simulink model "communicationCPU2_controller1"  (R2020a)
settings: Solver=FixedStepAuto  StartTime=0.0  StopTime=Inf  RelTol=1e-3  EnableMultiTasking=on
InitFcn:
  | Send_PSO_sample_time = 0.1;
undefined symbols (not defined in the file): C28x, CPU1, CPU2
libraries: c280xlib x10, c2837xDlib x3
settings Model: SimulationMode=external  ExtModeTrigDuration=8  Creator=Jason  LastModifiedBy=Jason
settings SolverCC: AutoInsertRateTranBlk=on
settings OptimizationCC: DefaultUnderspecifiedDataType=single  EnhancedBackFolding=on  PassReuseOutputArgsAs=Individual arguments  MaxStackSize=1024  OptimizeBlockOrder=speed  DifferentSizesBufferReuse=on  OptimizationCustomize=off  DenormalBehavior=FlushToZero  EfficientTunableParamExpr=on
settings DebuggingCC: ParameterTunabilityLossMsg=error
settings HardwareCC: ProdBitPerChar=16  ProdBitPerInt=16  ProdBitPerPointer=32  ProdBitPerSizeT=32  ProdBitPerPtrDiffT=32  ProdLargestAtomicInteger=Integer  ProdLargestAtomicFloat=None  ProdWordSize=16  ProdLongLongMode=on  ProdHWDeviceType=Texas Instruments->C2000
settings RTWCC: SystemTargetFile=ert.tlc  HardwareBoard=TI Delfino F28379D LaunchPad  TLCOptions=-aInlineSetEventsForThisBaseRateFcn=TLC_FALSE -aSuppressMultiTaskScheduler=TLC_FALSE -aRateBasedStepFcn=1  TemplateMakefile=ert_default_tmf  Toolchain=Texas Instruments Code Composer Studio (C2000)
settings CodeAppCC: ForceParamTrailComments=on  IgnoreCustomStorageClasses=off  OperatorAnnotations=on  SimulinkDataObjDesc=on  SFDataObjDesc=on  InsertBlockDesc=on
settings ERTTargetCC: TargetLangStandard=C99 (ISO)  CodeReplacementLibrary=TI C28x  SupportVariableSizeSignals=on  ExtModeStaticAllocSize=10000

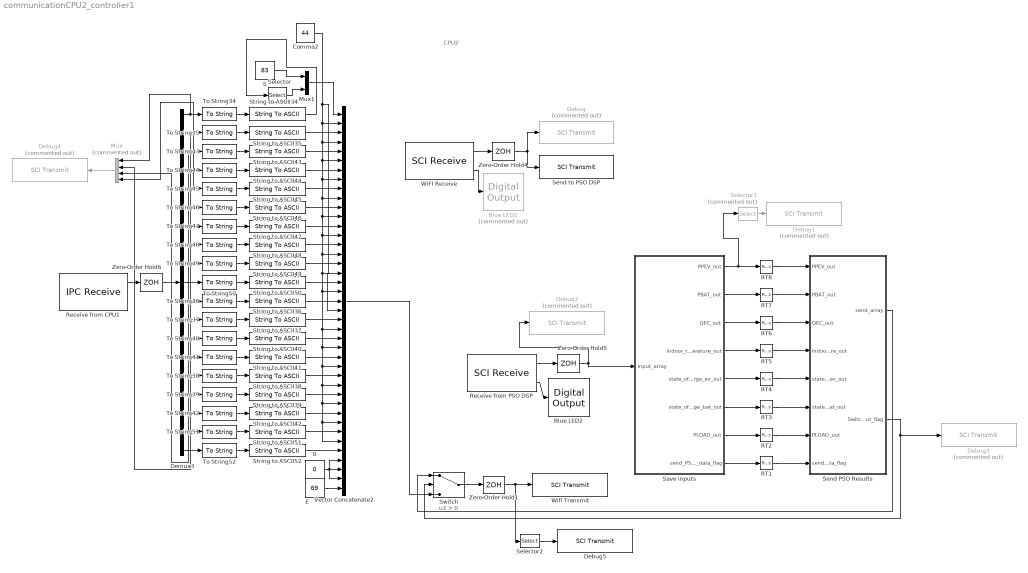
== system communicationCPU2_controller1 ==
  note: CPU2
  0 : Constant  Value=0  OutDataTypeStr=uint8  SampleTime=-1
  Blue LED1 : c2837xDlib/Digital Output  Commented=on  GPIO_Number=GPIO24~GPIO31  GPIO_Bit0=off  GPIO_BIT0_Toggle=off  GPIO_Bit1=off  GPIO_BIT1_Toggle=off  GPIO_Bit2=off  GPIO_BIT2_Toggle=off  GPIO_Bit3=off  GPIO_BIT3_Toggle=off  GPIO_Bit4=off  GPIO_BIT4_Toggle=off  GPIO_Bit5=off  GPIO_BIT5_Toggle=off  GPIO_Bit6=off  GPIO_BIT6_Toggle=off  GPIO_Bit7=on  GPIO_BIT7_Toggle=off
      settings: SourceProductBaseCode=TIC2000
  Blue LED2 : c2837xDlib/Digital Output  GPIO_Number=GPIO24~GPIO31  GPIO_Bit0=off  GPIO_BIT0_Toggle=off  GPIO_Bit1=off  GPIO_BIT1_Toggle=off  GPIO_Bit2=off  GPIO_BIT2_Toggle=off  GPIO_Bit3=off  GPIO_BIT3_Toggle=off  GPIO_Bit4=off  GPIO_BIT4_Toggle=off  GPIO_Bit5=off  GPIO_BIT5_Toggle=off  GPIO_Bit6=off  GPIO_BIT6_Toggle=off  GPIO_Bit7=on  GPIO_BIT7_Toggle=off
      settings: SourceProductBaseCode=TIC2000
  Comma2 : Constant  Value=44  OutDataTypeStr=uint8  SampleTime=-1
  Debug{,1..4} (5 alike) : c280xlib/SCI Transmit  Commented=on  sciModule=A  dataHead=''  dataTail=''  postInterrupt=off  numFifo=1
  Debug5 : c280xlib/SCI Transmit  sciModule=A  dataHead=''  dataTail=''  postInterrupt=off  numFifo=1
  Demux3 : Demux  Outputs=19
  E : Constant  Value=69  OutDataTypeStr=uint8  SampleTime=-1
  Mux : Mux  Commented=on
  Mux1 : Mux  Inputs=2
  RT{1..8} (8 alike) : RateTransition  OutPortSampleTime=Send_PSO_sample_time
  Receive from CPU1 : c2837xDlib/IPC Receive  blkParamProc=F2837x  SelectSource=C28x (CPU1/CPU2)  SelectChannel=0  DataType=single  DataLength=19  EnableBlocking=off  SampleTime=0.5
      settings: SourceProductBaseCode=TIC2000
  Receive from PSO DSP : c280xlib/SCI Receive  sciModule=B  dataHead=''  dataTail=''  dataType=uint8  dataDim=10  initValue=66  errOption=Output the last received value  errValue=0  sampleTime=0.005  outputStatus=on  postInterrupt=off  numFifo=1
      settings: SourceProductBaseCode=TIC2000
  S : Constant  Value=83  OutDataTypeStr=uint8  SampleTime=-1
  Save inputs : MATLAB Function  TreatAsAtomicUnit=on
  Selector : Selector  InputPortWidth=12  IndexOptions=Index vector (dialog)  Indices=[2:12]  OutputSizes=1
  Selector1 : Selector  Commented=on  InputPortWidth=500  IndexOptions=Index vector (dialog)  Indices=[481:500]  OutputSizes=1
  Selector2 : Selector  InputPortWidth=250  IndexOptions=Index vector (dialog)  Indices=[1:11]  OutputSizes=1
  Send PSO Results : MATLAB Function  TreatAsAtomicUnit=on
  Send to PSO DSP : c280xlib/SCI Transmit  sciModule=B  dataHead=''  dataTail=''  postInterrupt=off  numFifo=1
  String to ASCII{34..52} (19 alike) : StringToASCII  OutputVectorSize=12
  Switch : Switch  Criteria=u2 > Threshold
  To String{34..52} (19 alike) : ToString
  Vector Concatenate2 : Concatenate  NumInputs=41
  WiFI Receive : c280xlib/SCI Receive  sciModule=C  dataHead=''  dataTail=''  dataType=uint8  dataDim=11  initValue=50  errOption=Output the last received value  errValue=0  sampleTime=0.005  outputStatus=on  postInterrupt=off  numFifo=1
      settings: SourceProductBaseCode=TIC2000
  Wifi Transmit : c280xlib/SCI Transmit  sciModule=C  dataHead=''  dataTail=''  postInterrupt=off  numFifo=1
  Zero-Order Hold1 : ZeroOrderHold  SampleTime=0.4
  Zero-Order Hold4 : ZeroOrderHold  SampleTime=0.1
  Zero-Order Hold5 : ZeroOrderHold  SampleTime=0.05
  Zero-Order Hold6 : ZeroOrderHold  SampleTime=0.1
  wires:
  Demux3/2 -> Mux/2, To String35/1
  String to ASCII48/1 -> Vector Concatenate2/15
  To String39/1 -> String to ASCII39/1
  To String38/1 -> String to ASCII38/1
  String to ASCII39/1 -> Vector Concatenate2/31
  Demux3/17 -> To String42/1
  Demux3/16 -> To String39/1
  To String42/1 -> String to ASCII42/1
  Demux3/10 -> To String50/1
  Demux3/12 -> To String37/1
  Demux3/15 -> To String38/1
  String to ASCII35/1 -> Vector Concatenate2/3
  String to ASCII38/1 -> Vector Concatenate2/29
  String to ASCII42/1 -> Vector Concatenate2/33
  Demux3/14 -> To String41/1
  String to ASCII50/1 -> Vector Concatenate2/19
  String to ASCII44/1 -> Vector Concatenate2/7
  String to ASCII49/1 -> Vector Concatenate2/17
  String to ASCII40/1 -> Vector Concatenate2/25
  To String37/1 -> String to ASCII37/1
  To String36/1 -> String to ASCII36/1
  To String50/1 -> String to ASCII50/1
  String to ASCII46/1 -> Vector Concatenate2/11
  Demux3/8 -> To String48/1
  Demux3/7 -> To String47/1
  Demux3/6 -> To String46/1
  To String35/1 -> String to ASCII35/1
  To String47/1 -> String to ASCII47/1
  To String48/1 -> String to ASCII48/1
  String to ASCII36/1 -> Vector Concatenate2/21
  Demux3/5 -> Mux/4, To String45/1
  To String41/1 -> String to ASCII41/1
  Comma2/1 -> Vector Concatenate2/14, Vector Concatenate2/34, Vector Concatenate2/36, Vector Concatenate2/32, Vector Concatenate2/30, Vector Concatenate2/28, Vector Concatenate2/26, Vector Concatenate2/24, Vector Concatenate2/22, Vector Concatenate2/20, Vector Concatenate2/18, Vector Concatenate2/16, Vector Concatenate2/12, Vector Concatenate2/10, Vector Concatenate2/8, Vector Concatenate2/6, Vector Concatenate2/4, Vector Concatenate2/2
  String to ASCII47/1 -> Vector Concatenate2/13
  String to ASCII43/1 -> Vector Concatenate2/5
  To String45/1 -> String to ASCII45/1
  To String49/1 -> String to ASCII49/1
  To String46/1 -> String to ASCII46/1
  Demux3/11 -> To String36/1
  Demux3/3 -> Mux/3, To String43/1
  String to ASCII41/1 -> Vector Concatenate2/27
  To String44/1 -> String to ASCII44/1
  Demux3/13 -> To String40/1
  Demux3/1 -> Mux/1, To String34/1
  String to ASCII37/1 -> Vector Concatenate2/23
  Demux3/9 -> To String49/1
  String to ASCII45/1 -> Vector Concatenate2/9
  To String43/1 -> String to ASCII43/1
  Demux3/4 -> To String44/1
  To String40/1 -> String to ASCII40/1
  To String34/1 -> String to ASCII34/1
  To String51/1 -> String to ASCII51/1
  String to ASCII51/1 -> Vector Concatenate2/35
  Demux3/18 -> To String51/1
  To String52/1 -> String to ASCII52/1
  Demux3/19 -> To String52/1
  String to ASCII52/1 -> Vector Concatenate2/37
  0/1 -> Vector Concatenate2/38, Vector Concatenate2/40, Vector Concatenate2/39
  E/1 -> Vector Concatenate2/41
  Selector/1 -> Mux1/2
  S/1 -> Mux1/1
  String to ASCII34/1 -> Selector/1
  Mux1/1 -> Vector Concatenate2/1
  Vector Concatenate2/1 -> Switch/3
  WiFI Receive/1 -> Zero-Order Hold4/1
  Zero-Order Hold4/1 -> Debug/1, Send to PSO DSP/1
  Receive from PSO DSP/1 -> Zero-Order Hold5/1
  Zero-Order Hold5/1 -> Save inputs/1(input_array), Debug2/1
  Receive from CPU1/1 -> Zero-Order Hold6/1
  Zero-Order Hold6/1 -> Demux3/1
  Receive from PSO DSP/2 -> Blue LED2/1
  WiFI Receive/2 -> Blue LED1/1
  Save inputs/1(PPEV_out) -> RT8/1, Selector1/1
  Switch/1 -> Zero-Order Hold1/1
  Send PSO Results/1(send_array) -> Switch/1
  Send PSO Results/2(Switch_output_flag) -> Debug3/1, Switch/2
  Selector1/1 -> Debug1/1
  Save inputs/7(PLOAD_out) -> RT2/1
  Save inputs/8(send_PSO_data_flag) -> RT1/1
  RT2/1 -> Send PSO Results/7(PLOAD_out)
  Save inputs/6(state_of_charge_bat_out) -> RT3/1
  RT3/1 -> Send PSO Results/6(state_of_charge_bat_out)
  Save inputs/5(state_of_charge_ev_out) -> RT4/1
  RT4/1 -> Send PSO Results/5(state_of_charge_ev_out)
  Save inputs/4(indoor_temperature_out) -> RT5/1
  RT5/1 -> Send PSO Results/4(indoor_temperature_out)
  Save inputs/3(QEC_out) -> RT6/1
  RT6/1 -> Send PSO Results/3(QEC_out)
  Save inputs/2(PBAT_out) -> RT7/1
  RT7/1 -> Send PSO Results/2(PBAT_out)
  RT8/1 -> Send PSO Results/1(PPEV_out)
  RT1/1 -> Send PSO Results/8(send_PSO_data_flag)
  Zero-Order Hold1/1 -> Selector2/1, Wifi Transmit/1
  Mux/1 -> Debug4/1
  Selector2/1 -> Debug5/1

== matlab function communicationCPU2_controller1/Send PSO Results ==
  data: PPEV_out input; send_array output uint8 size=1 250; PBAT_out input; QEC_out input; indoor_temperature_out input; state_of_charge_ev_out input; state_of_charge_bat_out input; PLOAD_out input; Switch_output_flag output; send_PSO_data_flag input
function [send_array,Switch_output_flag] = send_PSO_data(PPEV_out,PBAT_out,QEC_out,indoor_temperature_out,state_of_charge_ev_out,state_of_charge_bat_out,PLOAD_out,send_PSO_data_flag)


persistent send_arr counter flag start_flag

if isempty(send_arr)
    send_arr = uint8(zeros(1,250));
    counter = single(0);
    %     flag = single(0);
    start_flag = single(0);
end

if send_PSO_data_flag == 1 && start_flag == 0
    counter = single(1);
    start_flag = single(1);
end

if start_flag == 1
    
    if counter == single(1)
        send_arr(1:250) = PPEV_out(1:250);
        send_arr(1) = 83; %S
        send_arr(2) = 90; %Z
        send_arr(9) = 97; %a
        send_arr(250) = 69; %E
    elseif counter == single(15)
        send_arr(1:250) = PPEV_out(251:500);
        send_arr(9) = 98; %b
        send_arr(250) = 69; %E
        
    elseif counter == single(30)
        send_arr(1:250) = PBAT_out(1:250);
        send_arr(1) = 83; %S
        send_arr(2) = 79; %O
        send_arr(9) = 99; %c
        send_arr(250) = 69; %E
    elseif counter == single(45)
        send_arr(1:250) = PBAT_out(251:500);
        send_arr(9) = 100; %d
        send_arr(250) = 69; %E
        
    elseif counter == single(60)
        send_arr(1:250) = QEC_out(1:250);
        send_arr(1) = 83; %S
        send_arr(2) = 79; %O
        send_arr(9) = 101; %e
        send_arr(250) = 69; %E
    elseif counter == single(75)
        send_arr(1:250) = QEC_out(251:500);
        send_arr(9) = 102; %f
        send_arr(250) = 69; %E
        
    elseif counter == single(90)
        send_arr(1:250) = indoor_temperature_out(1:250);
        send_arr(1) = 83; %S
        send_arr(2) = 79; %O
        send_arr(9) = 103; %g
        send_arr(250) = 69; %E
    elseif counter == single(105)
        send_arr(1:250) = indoor_temperature_out(251:500);
        send_arr(9) = 104; %h
        send_arr(250) = 69; %E
        
    elseif counter == single(120)
        send_arr(1:250) = state_of_charge_ev_out(1:250);
        send_arr(1) = 83; %S
        send_arr(2) = 79; %O
        send_arr(9) = 105; %i
        send_arr(250) = 69; %E
    elseif counter == single(135)
        send_arr(1:250) = state_of_charge_ev_out(251:500);
        send_arr(9) = 106; %j
        send_arr(250) = 69; %E
        
    elseif counter == single(150)
        send_arr(1:250) = state_of_charge_bat_out(1:250);
        send_arr(1) = 83; %S
        send_arr(2) = 79; %O
        send_arr(9) = 107; %k
        send_arr(250) = 69; %E
    elseif counter == single(165)
        send_arr(1:250) = state_of_charge_bat_out(251:500);
        send_arr(9) = 108; %l
        send_arr(250) = 69; %E
        
    elseif counter == single(180)
        send_arr(1:250) = PLOAD_out(1:250);
        send_arr(1) = 83; %S
        send_arr(2) = 79; %O
        send_arr(9) = 109; %m
        send_arr(250) = 69; %E
    elseif counter == single(195)
        send_arr(1:250) = PLOAD_out(251:500);
        send_arr(9) = 110; %n
        send_arr(250) = 69; %E
    end
    
    
    
    if counter >=1 && counter <210
        flag = single(1);
    else
        flag = single(0);
    end
    
    
    counter = counter + 1;
    
    
    if counter == 5000
        counter = single(1);
    end
else
    flag = single(0);
end

send_array = send_arr(1:250);
Switch_output_flag = flag;

== matlab function communicationCPU2_controller1/Save inputs ==
  data: input_array input; PPEV_out output; PBAT_out output; QEC_out output; indoor_temperature_out output; state_of_charge_ev_out output; state_of_charge_bat_out output; PLOAD_out output; send_PSO_data_flag output
function [PPEV_out,PBAT_out,QEC_out,indoor_temperature_out,state_of_charge_ev_out,state_of_charge_bat_out,PLOAD_out,send_PSO_data_flag]= save_inputs(input_array)

    
%    output_array_temp = single([1111111 debug_array 2222222 debug_array 3333333 debug_array 4444444 debug_array ...
%         5555555 debug_array 6666666 debug_array 7777777 debug_array]);
        
        
persistent PPEV PBAT QEC indoor_temperature state_of_charge_ev state_of_charge_bat PLOAD counter mode flag
% PPEV_out,PBAT_out,QEC_out,indoor_temperature_out,state_of_charge_ev_out,state_of_charge_bat_out,PLOAD_out

if isempty(PPEV)
    PPEV = uint8(zeros(1,500));
    PBAT = uint8(zeros(1,500));
    QEC = uint8(zeros(1,500));
    indoor_temperature = uint8(zeros(1,500));
    state_of_charge_ev = uint8(zeros(1,500));
    state_of_charge_bat = uint8(zeros(1,500));
    PLOAD = uint8(zeros(1,500));
    counter = single(0);
    mode = single(0);
    flag = single(0);
end



if input_array(1:10) == [49 49 49 49 49 49 49 0 0 44]'   %1111111
    counter = single(1);
    PPEV(1:10) = input_array(1:10);
    mode = single(1);
    counter = counter + 10;
elseif input_array(1:10) == [50 50 50 50 50 50 50 0 0 44]'
    counter = single(1);
    PBAT(1:10) = input_array(1:10);
    mode = single(2);
    counter = counter + 10;
elseif input_array(1:10) == [51 51 51 51 51 51 51 0 0 44]'
    counter = single(1);
    QEC(1:10) = input_array(1:10);
    mode = single(3);
    counter = counter + 10;
elseif input_array(1:10) == [52 52 52 52 52 52 52 0 0 44]'
    counter = single(1);
    indoor_temperature(1:10) = input_array(1:10);
    mode = single(4);
    counter = counter + 10;
elseif input_array(1:10) == [53 53 53 53 53 53 53 0 0 44]'
    counter = single(1);
    state_of_charge_ev(1:10) = input_array(1:10);
    mode = single(5);
    counter = counter + 10;
elseif input_array(1:10) == [54 54 54 54 54 54 54 0 0 44]'
    counter = single(1);
    state_of_charge_bat(1:10) = input_array(1:10);
    mode = single(6);
    counter = counter + 10;
elseif input_array(1:10) == [55 55 55 55 55 55 55 0 0 44]'
    counter = single(1);
    PLOAD(1:10) = input_array(1:10);
    mode = single(7);
    counter = counter + 10;
elseif mode == 1 && input_array(10) == ','
    PPEV(counter:counter+9) = input_array(1:10);
    counter = counter + 10;
elseif mode == 2 && input_array(10) == ','
    PBAT(counter:counter+9) = input_array(1:10);
    counter = counter + 10;
elseif mode == 3 && input_array(10) == ','
    QEC(counter:counter+9) = input_array(1:10);
    counter = counter + 10;
elseif mode == 4 && input_array(10) == ','
    indoor_temperature(counter:counter+9) = input_array(1:10);
    counter = counter + 10;
elseif mode == 5 && input_array(10) == ','
    state_of_charge_ev(counter:counter+9) = input_array(1:10);
    counter = counter + 10;
elseif mode == 6 && input_array(10) == ','
    state_of_charge_bat(counter:counter+9) = input_array(1:10);
    counter = counter + 10;
elseif mode == 7 && input_array(10) == ','
    PLOAD(counter:counter+9) = input_array(1:10);
    counter = counter + 10;
    if counter == 501
%         PPEV(1:10) = [111 111 111 111 111 111 111 111 111 111]';
        flag = single(1);
    end
else
    flag = single(0);
end

PPEV_out = PPEV;
PBAT_out = PBAT;
QEC_out = QEC;
indoor_temperature_out = indoor_temperature;
state_of_charge_ev_out = state_of_charge_ev;
state_of_charge_bat_out = state_of_charge_bat;
PLOAD_out = PLOAD;
send_PSO_data_flag = flag;
